simulink model "hexAeroCoefficientsModel"  (R2024a)
settings: configuration reference "standardSILConfiguraitonParams" (kept outside this file)
undefined symbols (not defined in the file): alphaBkpts_rad, C_D, C_L
libraries: aerolibtransform2 x1
settings Model: Creator=GTAR  LastModifiedBy=jerem
settings ConfigSetRef: SourceName=standardSILConfiguraitonParams  SourceLocation=Base Workspace

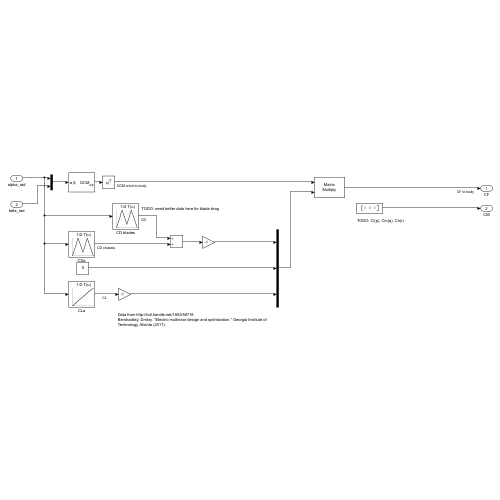
[thumbnail: Simulink's stored preview of the top-level diagram]
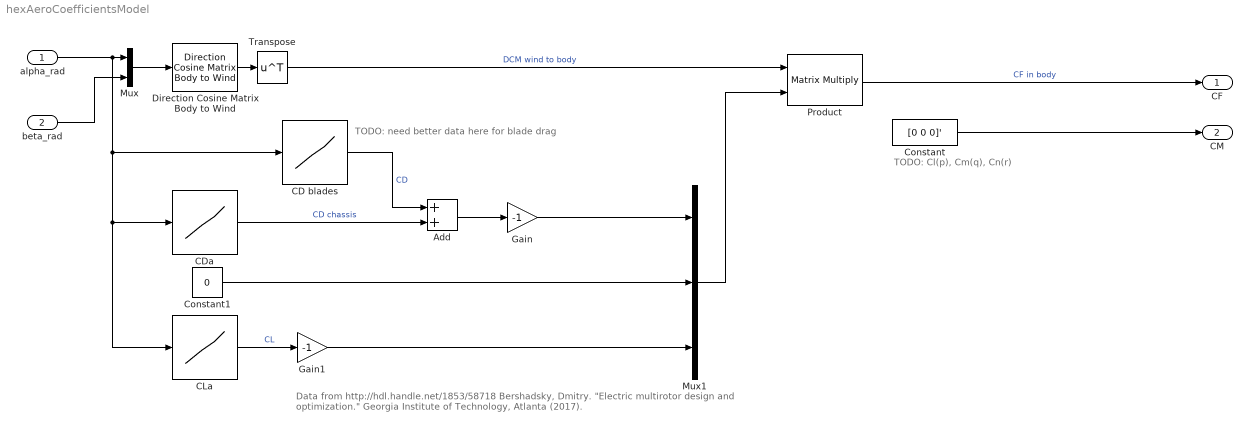
== system hexAeroCoefficientsModel ==
  note: TODO: Cl(p), Cm(q), Cn(r)
  note: TODO: need better data here for blade drag
  note: Data from http://hdl.handle.net/1853/58718
      | Bershadsky, Dmitry. "Electric multirotor design and optimization." Georgia Institute of Technology, Atlanta (2017).
  alpha_rad : Inport
  beta_rad : Inport  Port=2
  Add : Sum
  CD blades : Lookup_n-D  NumberOfTableDimensions=1  BreakpointsForDimension1=alphaBkpts_rad  Table=C_D  InternalRulePriority=Speed  RndMeth=Simplest
  CDa : Lookup_n-D  NumberOfTableDimensions=1  BreakpointsForDimension1=alphaBkpts_rad  Table=C_D  InternalRulePriority=Speed  RndMeth=Simplest
  CLa : Lookup_n-D  NumberOfTableDimensions=1  BreakpointsForDimension1=alphaBkpts_rad  Table=C_L  InternalRulePriority=Speed  RndMeth=Simplest
  Constant : Constant  Value=[0 0 0]'
  Constant1 : Constant  Value=0
  Direction Cosine Matrix Body to Wind : aerolibtransform2/Direction Cosine Matrix Body to Wind
  Gain : Gain  Gain=-1
  Gain1 : Gain  Gain=-1
  Mux : Mux  Inputs=2
  Mux1 : Mux  Inputs=3
  Product : Product  Multiplication=Matrix(*)
  Transpose : Math  Operator=transpose
  CF : Outport
  CM : Outport  Port=2
  wires:
  Product/1 -> CF/1  "CF in body"
  beta_rad/1 -> Mux/2
  alpha_rad/1 -> CD blades/1, CDa/1, CLa/1, Mux/1
  Constant/1 -> CM/1
  Direction Cosine Matrix Body to Wind/1 -> Transpose/1
  Mux/1 -> Direction Cosine Matrix Body to Wind/1
  Transpose/1 -> Product/1  "DCM wind to body"
  CDa/1 -> Add/2  "CD chassis"
  CLa/1 -> Gain1/1  "CL"
  Constant1/1 -> Mux1/2
  Mux1/1 -> Product/2
  Gain/1 -> Mux1/1
  Gain1/1 -> Mux1/3
  Add/1 -> Gain/1
  CD blades/1 -> Add/1  "CD"
